simulink model "PP3"  (R2023a)
settings: Solver=VariableStepAuto  StartTime=0.0  StopTime=10.0  RelTol=1e-3
values from neighbouring files (symbols this model uses):
  a1 = 290    [PARAMETROS.m]    (also in signal.m)
  a2 = 59    [PARAMETROS.m]    (also in signal.m)
  b1 = 1000    [PARAMETROS.m]    (also in signal.m)
  c1 = 16182    [PARAMETROS.m]    (also in signal.m)
  c2 = 19000    [PARAMETROS.m]    (also in signal.m)
settings Model: Creator=escor  LastModifiedBy=cash
settings OptimizationCC: ReuseModelBlockBuffer=off

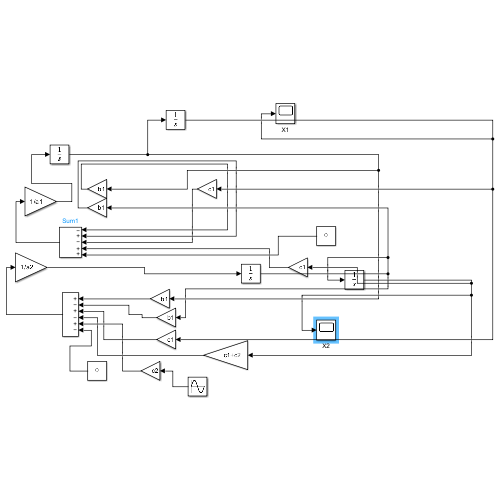
[thumbnail: Simulink's stored preview of the top-level diagram]
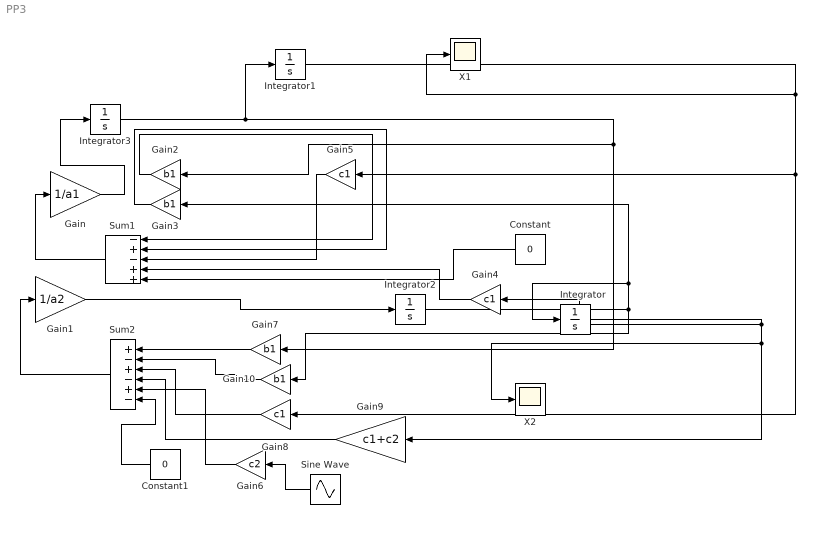
== system PP3 ==
  Constant : Constant  Value=0
  Constant1 : Constant  Value=0
  Gain : Gain  Gain=1/a1
  Gain1 : Gain  Gain=1/a2
  Gain{2..3,7,10} (4 alike) : Gain  Gain=b1
  Gain4 : Gain  Gain=c1
  Gain5 : Gain  Gain=c1
  Gain6 : Gain  Gain=c2
  Gain8 : Gain  Gain=c1
  Gain9 : Gain  Gain=c1+c2
  Integrator{,1..3} (4 alike) : Integrator
  Sine Wave : Sin  Amplitude=0.05  Frequency=0.5*pi  SampleTime=0
  Sum1 : Sum  Inputs=-+-++
  Sum2 : Sum  Inputs=+-+-+-
  X1 : Scope
  X2 : Scope
  wires:
  Sum2/1 -> Gain1/1
  Gain7/1 -> Sum2/1
  Sum1/1 -> Gain/1
  Integrator3/1 -> Gain7/1, Gain2/1, Integrator1/1
  Gain5/1 -> Sum1/3
  Gain9/1 -> Sum2/4
  Constant1/1 -> Sum2/6
  Gain4/1 -> Sum1/4
  Gain6/1 -> Sum2/5
  Sine Wave/1 -> Gain6/1
  Integrator2/1 -> Integrator/1, Gain3/1, Gain10/1
  Constant/1 -> Sum1/5
  Gain10/1 -> Sum2/2
  Integrator/1 -> X2/1, Gain9/1, Gain4/1
  Gain/1 -> Integrator3/1
  Gain8/1 -> Sum2/3
  Gain1/1 -> Integrator2/1
  Gain2/1 -> Sum1/1
  Gain3/1 -> Sum1/2
  Integrator1/1 -> X1/1, Gain8/1, Gain5/1
